simulink model "switching_graphs"  (R2021a)
settings: Solver=VariableStepAuto  StartTime=0.0  StopTime=50/80e3  FixedStep=1e-7  MaxStep=1e-7  MinStep=1e-9  RelTol=1e-7
undefined symbols (not defined in the file or in its folder): L, R
libraries: spsSeriesRLCBranchLib x2, spsControlledVoltageSourceLib x1, spsTriangleGeneratorLib x1, spsVoltageMeasurementLib x1, spspowerguiLib x1
settings Model: Creator=enes_  LastModifiedBy=enes_

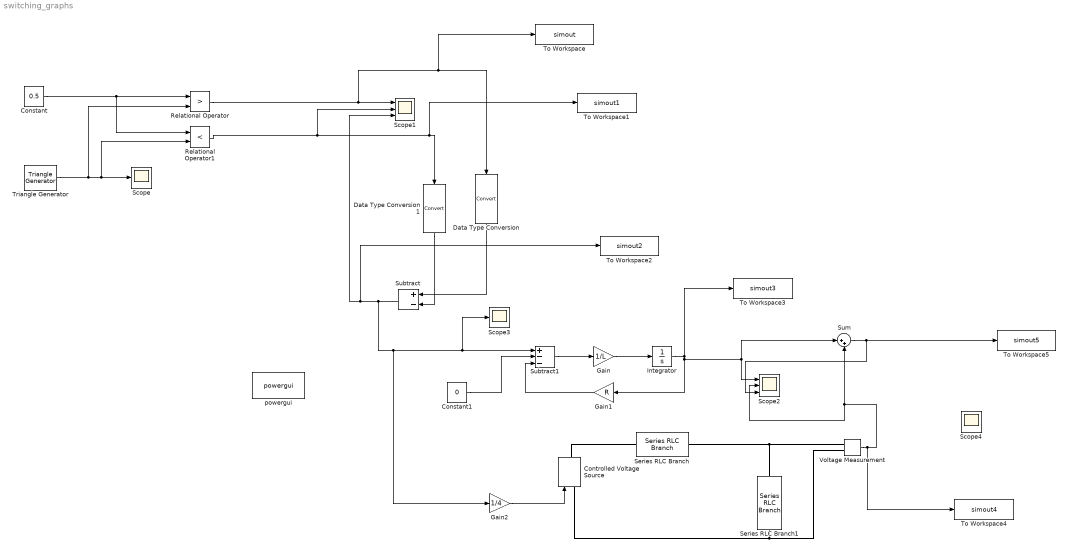
== system switching_graphs ==
  Constant : Constant  Value=0.5
  Constant1 : Constant  Value=0
  Controlled Voltage Source : spsControlledVoltageSourceLib/Controlled Voltage Source  Initialize=on  Source_Type=AC  Amplitude=0  Phase=0  Frequency=0  Measurements=None
  Data Type Conversion : DataTypeConversion
  Data Type Conversion1 : DataTypeConversion
  Gain : Gain  Gain=1/L
  Gain1 : Gain  Gain=R
  Gain2 : Gain  Gain=1/4
  Integrator : Integrator  InitialCondition=4.88
  Relational Operator : RelationalOperator  Operator=>  OutDataTypeStr=boolean  RndMeth=Simplest
  Relational Operator1 : RelationalOperator  Operator=<  OutDataTypeStr=boolean  RndMeth=Simplest
  Scope : Scope
  Scope1 : Scope  NumInputPorts=3
  Scope2 : Scope  NumInputPorts=3
  Scope3 : Scope
  Scope4 : Scope
  Series RLC Branch : spsSeriesRLCBranchLib/Series RLC Branch  LConnTagsString=__new0  RConnTagsString=__new0  BranchType=LC  Resistance=1  Inductance=100e-6  SetiL0=off  InitialCurrent=0  Capacitance=3.9579e-08  Setx0=off  InitialVoltage=0  Measurements=None
  Series RLC Branch1 : spsSeriesRLCBranchLib/Series RLC Branch  LConnTagsString=__new0  RConnTagsString=__new0  BranchType=R  Resistance=1  Inductance=100e-6  SetiL0=off  InitialCurrent=0  Capacitance=3.9579e-08  Setx0=off  InitialVoltage=0  Measurements=None
  Subtract : Sum  Inputs=+-
  Subtract1 : Sum  Inputs=+--
  Sum : Sum  Inputs=|++
  To Workspace : ToWorkspace  VariableName=simout  SaveFormat=Timeseries  SampleTime=-1
  To Workspace1 : ToWorkspace  VariableName=simout1  SaveFormat=Timeseries  SampleTime=-1
  To Workspace2 : ToWorkspace  VariableName=simout2  SaveFormat=Timeseries  SampleTime=-1
  To Workspace3 : ToWorkspace  VariableName=simout3  SaveFormat=Timeseries  SampleTime=-1
  To Workspace4 : ToWorkspace  VariableName=simout4  SaveFormat=Timeseries  SampleTime=-1
  To Workspace5 : ToWorkspace  VariableName=simout5  SaveFormat=Timeseries  SampleTime=-1
  Triangle Generator : spsTriangleGeneratorLib/Triangle Generator  Freq=80e3  Phase=0  Ts=1e-8
  Voltage Measurement : spsVoltageMeasurementLib/Voltage Measurement  PhasorSimulation=off  OutputType=Complex  PSBequivalent=0
  powergui : spspowerguiLib/powergui  Priority=1  SimulationMode=Continuous  SampleTime=50e-6  frequency=60  Iterations=50  frequencyindice=0  Pbase=100e6  ErrMax=1e-4  UnitsV=kV  UnitsW=MW  buscounter=0  FunctionMessages=off  echomessages=off  EnableUseOfTLC=off  CurrentSourceSwitches=off  DisableSnubberDevices=off  DisableRonSwitches=off  DisableVfSwitches=off  DisplayEquations=off  AutomaticDiscreteSolvers=off  SolverType=Tustin/Backward Euler (TBE)  Interpol=off  ExternalGateDelay=off  methode=off  Ts=100  x0status=blocks  SPID=on  SwTol=0  HookPort=off  NonlinearTolerance=1e-4  nMaxIteration=100  ContinueOnMaxIteration=off  RestoreLinks=warning  ResistiveCurrentMeasurement=off  Frange=[0:2:500]  Ylog=off  Xlog=on  ShowGrid=off  save=off  variable=ZData  structure=0  ZoomFFT=off  StartTime=0.0  cycles=1  DisplayStyle=1  fundamental=60  FreqAxis=off  MaxFrequency=1000  frequencyindicesteady=1  RmsSteady=1  display=off
  wires:
  Triangle Generator/1 -> Relational Operator/2, Relational Operator1/2, Scope/1
  Constant/1 -> Relational Operator1/1, Relational Operator/1
  Relational Operator/1 -> To Workspace/1, Data Type Conversion/1, Scope1/1
  Relational Operator1/1 -> To Workspace1/1, Data Type Conversion1/1, Scope1/2
  Subtract/1 -> Gain2/1, Scope3/1, Subtract1/1, To Workspace2/1, Scope1/3
  Data Type Conversion/1 -> Subtract/1
  Data Type Conversion1/1 -> Subtract/2
  Constant1/1 -> Subtract1/2
  Subtract1/1 -> Gain/1
  Gain/1 -> Integrator/1
  Gain1/1 -> Subtract1/3
  Integrator/1 -> Sum/1, Scope2/1, Gain1/1, To Workspace3/1
  Gain2/1 -> Controlled Voltage Source/1
  Sum/1 -> Scope2/3, To Workspace5/1
  Voltage Measurement/1 -> To Workspace4/1, Sum/2, Scope2/2
  connections:
  Series RLC Branch/LConn1 -- Controlled Voltage Source/RConn1
  Controlled Voltage Source/LConn1 -- Voltage Measurement/LConn2 -- Series RLC Branch1/RConn1
  Series RLC Branch/RConn1 -- Series RLC Branch1/LConn1 -- Voltage Measurement/LConn1
